simulink model "Plant_C3"  (R2023a)
settings: Solver=ode45  StartTime=0.0  StopTime=10000  RelTol=1e-2  EnableMultiTasking=on
values from neighbouring files (symbols this model uses):
  alfa = [alfaa alfab alfac alfad alfae alfaf]    [ChemBenchData.m]    (also in dati.m)
  H3 = [Hr3;He3*ones(Ne3,1);Hf3;Ha3*ones(Na3,1);Hc3]    [ChemBenchData.m]    (also in dati.m)
  N3 = Na3+Ne3+3    (= 19)    [ChemBenchData.m]    (also in dati.m = 9)
  Na3 = 8    [ChemBenchData.m]    (also in dati.m = 3)
  Ne3 = 8    [ChemBenchData.m]    (also in dati.m = 3)
  V3 = 282    [ChemBenchData.m]    (also in dati.m)
  x3a = zeros(N3,1)    [ChemBenchData.m]    (also in dati.m)
  x3b = zeros(N3,1)    [ChemBenchData.m]    (also in dati.m)
  x3c = zeros(N3,1)    [ChemBenchData.m]    (also in dati.m)
undefined symbols (not defined in the file or in its folder): colonna3, somma
settings Model: Creator=scattolini  LastModifiedBy=laura
settings SolverCC: AlgebraicLoopSolver=TrustRegion
settings DataIOCC: LimitDataPoints=on  SaveFormat=Array  SignalLoggingSaveFormat=ModelDataLogs  ReturnWorkspaceOutputs=off
settings OptimizationCC: BlockReduction=off  DefaultParameterBehavior=Inlined  InlineInvariantSignals=on  BufferReuse=off  ExpressionDepthLimit=2147483647  InitFltsAndDblsToZero=on  LifeSpan=inf
settings DebuggingCC: SaveWithParameterizedLinksMsg=none  UnderspecifiedInitializationDetection=Classic  MergeDetectMultiDrivingBlocksExec=none  SignalResolutionControl=TryResolveAllWithWarning  SolverPrmCheckMsg=warning  MultiTaskDSMMsg=warning  MultiTaskCondExecSysMsg=none  FcnCallInpInsideContextMsg=warning  UnconnectedInputMsg=warning  UnconnectedOutputMsg=warning  UnconnectedLineMsg=warning  StateNameClashWarn=warning  SFUnexpectedBacktrackingDiag=warning  SFNoUnconditionalDefaultTransitionDiag=warning  SFExecutionAtInitializationDiag=none  ArithmeticOperatorsInVariantConditions=warning
settings HardwareCC: ProdBitPerPointer=32  ProdBitPerSizeT=32  ProdBitPerPtrDiffT=32  ProdLargestAtomicFloat=None  ProdIntDivRoundTo=Undefined  ProdEndianess=Unspecified  ProdWordSize=32  ProdHWDeviceType=32-bit Generic
settings ModelReferenceCC: EnableRefExpFcnMdlSchedulingChecks=on  PropagateSignalLabelsOutOfModel=off
settings RTWCC: DLArmComputeVersion=19.05
settings CodeAppCC: StateflowObjectComments=on
settings GRTTargetCC: TargetFcnLib=ansi_tfl_tmw.mat  TargetLangStandard=C89/C90 (ANSI)  CombineOutputUpdateFcns=off  GRTInterface=on
settings ConfigComp: CovMetricSettings=dw  CovSaveCumulativeToWorkspaceVar=on  CovSaveSingleToWorkspaceVar=on

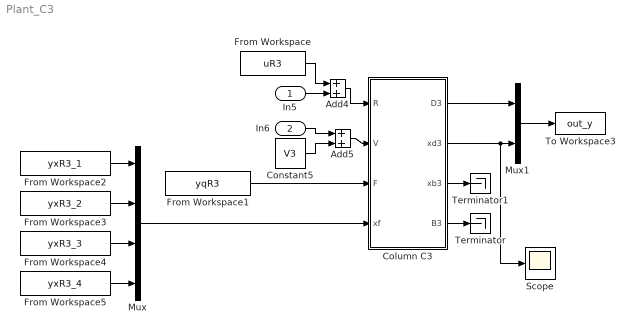
== system Plant_C3 ==
  In5 : Inport
  In6 : Inport  Port=2
  Add4 : Sum
  Add5 : Sum
  Column C3 : Subsystem
  Constant5 : Constant  Value=V3
  From Workspace : FromWorkspace  VariableName=uR3  SampleTime=-1
  From Workspace1 : FromWorkspace  VariableName=yqR3  SampleTime=-1
  From Workspace2 : FromWorkspace  VariableName=yxR3_1  SampleTime=-1
  From Workspace3 : FromWorkspace  VariableName=yxR3_2  SampleTime=-1
  From Workspace4 : FromWorkspace  VariableName=yxR3_3  SampleTime=-1
  From Workspace5 : FromWorkspace  VariableName=yxR3_4  SampleTime=-1
  Mux : Mux
  Mux1 : Mux  Inputs=2
  Scope : Scope
  Terminator : Terminator
  Terminator1 : Terminator
  To Workspace3 : ToWorkspace  VariableName=out_y  SampleTime=1
  wires:
  Column C3/2(xd3) -> Scope/1, Mux1/2
  Column C3/1(D3) -> Mux1/1
  From Workspace/1 -> Add4/1
  Add5/1 -> Column C3/2(V)
  Constant5/1 -> Add5/2
  In6/1 -> Add5/1
  In5/1 -> Add4/2
  Column C3/4(B3) -> Terminator/1
  Add4/1 -> Column C3/1(R)
  Mux1/1 -> To Workspace3/1
  From Workspace2/1 -> Mux/1
  From Workspace3/1 -> Mux/2
  From Workspace4/1 -> Mux/3
  From Workspace5/1 -> Mux/4
  From Workspace1/1 -> Column C3/3(F)
  Mux/1 -> Column C3/4(xf)
  Column C3/3(xb3) -> Terminator1/1

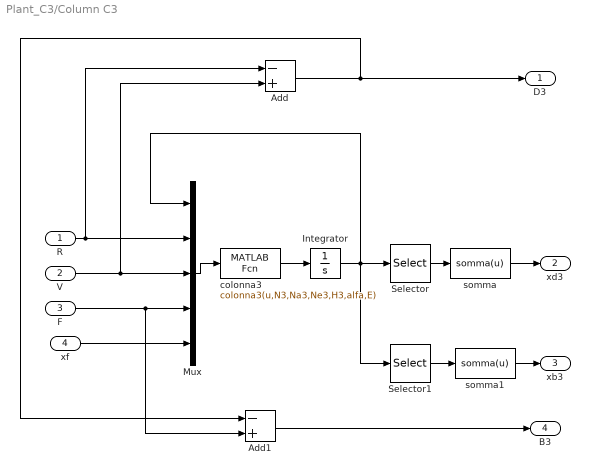
== system Plant_C3/Column C3 ==
  R : Inport
  V : Inport  Port=2
  F : Inport  Port=3
  xf : Inport  Port=4
  Add : Sum  Inputs=-+
  Add1 : Sum  Inputs=-+
  Integrator : Integrator  InitialCondition=[x3a;x3b;x3c]
  Mux : Mux  Inputs=5
  Selector : Selector  InputPortWidth=N3*3  IndexOptions=Index vector (dialog)  Indices=[N3 2*N3 3*N3]  OutputSizes=1
  Selector1 : Selector  InputPortWidth=N3*3  IndexOptions=Index vector (dialog)  Indices=[1 N3+1 2*N3+1]  OutputSizes=1
  colonna3 : MATLABFcn  MATLABFcn=colonna3(u,N3,Na3,Ne3,H3,alfa,E)  OutputDimensions=N3*3
  somma : MATLABFcn  MATLABFcn=somma(u)  OutputDimensions=4
  somma1 : MATLABFcn  MATLABFcn=somma(u)  OutputDimensions=4
  D3 : Outport
  xd3 : Outport  Port=2
  xb3 : Outport  Port=3
  B3 : Outport  Port=4
  wires:
  Mux/1 -> colonna3/1
  colonna3/1 -> Integrator/1
  Integrator/1 -> Selector/1, Mux/1, Selector1/1
  R/1 -> Mux/2, Add/1
  V/1 -> Mux/3, Add/2
  F/1 -> Mux/4, Add1/2
  xf/1 -> Mux/5
  Selector/1 -> somma/1
  somma/1 -> xd3/1
  Selector1/1 -> somma1/1
  somma1/1 -> xb3/1
  Add/1 -> D3/1, Add1/1
  Add1/1 -> B3/1
